simulink model "NL_valve"  (Simulink 7.8)
settings: Solver=ode45  StartTime=0.0  StopTime=time_span  RelTol=1e-3
values from neighbouring files (symbols this model uses):
  Cm = 5    [MSA_Controller.m]    (also in MSA_Controller_NL_valve.m = 1)
  par = [0.1,0.1,0.1]    [MSA_Controller.m]    (also in MSA_Controller_NL_valve.m = [0.1,0.1])
  samp_time = p.simulation.samp_time    [MSA_Controller.m]    (also in MSA_Controller_NL_valve.m)
libraries: simulink x1, simulink_need_slupdate x1
settings Model: Creator=KushalSahare  LastModifiedBy=KushalSahare

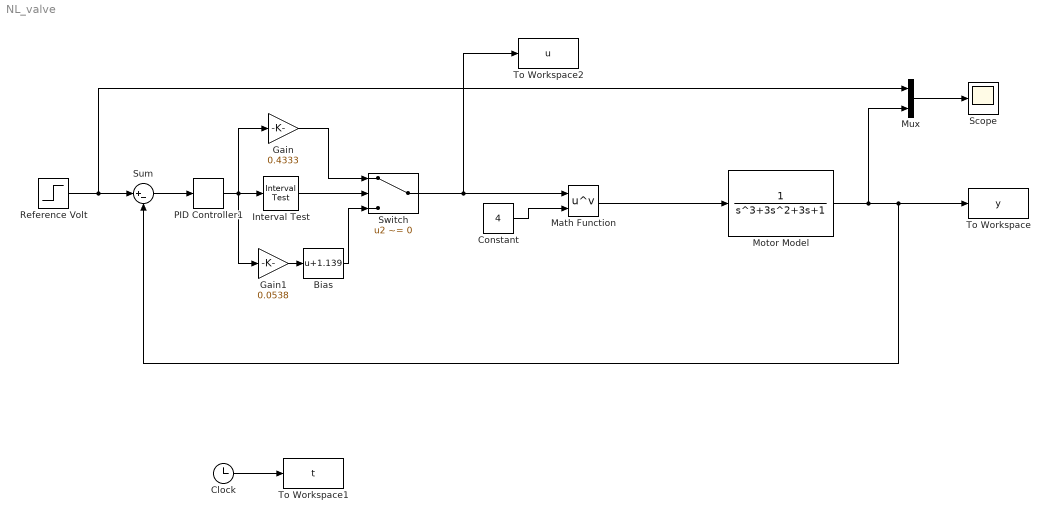
== system NL_valve ==
  Bias : Bias  Bias=1.139
  Clock : Clock
  Constant : Constant  Value=4
  Gain : Gain  Gain=0.4333
  Gain1 : Gain  Gain=0.0538
  Interval Test : simulink/Logic and Bit Operations/Interval Test  IntervalClosedRight=on  uplimit=3  IntervalClosedLeft=on  lowlimit=0  OutDataTypeStr=boolean
  Math Function : Math  Operator=pow  SaturateOnIntegerOverflow=on
  Motor Model : TransferFcn  Numerator=1  Denominator=[1, 3, 3, 1]
  Mux : Mux  Inputs=2
  PID Controller1 : simulink_need_slupdate/PID Controller  P=par(1)  I=par(2)  D=par(3)
  Reference Volt : Step  Time=0  After=Cm  SampleTime=0
  Scope : Scope
  Sum : Sum  Inputs=|+-
  Switch : Switch  Criteria=u2 ~= 0
  To Workspace : ToWorkspace  VariableName=y  SampleTime=samp_time  SaveFormat=Array
  To Workspace1 : ToWorkspace  VariableName=t  SampleTime=samp_time  SaveFormat=Array
  To Workspace2 : ToWorkspace  VariableName=u  SampleTime=samp_time  SaveFormat=Array
  wires:
  Motor Model/1 -> Sum/2, To Workspace/1, Mux/2
  Sum/1 -> PID Controller1/1
  PID Controller1/1 -> Interval Test/1, Gain/1, Gain1/1
  Reference Volt/1 -> Sum/1, Mux/1
  Constant/1 -> Math Function/2
  Math Function/1 -> Motor Model/1
  Clock/1 -> To Workspace1/1
  Mux/1 -> Scope/1
  Interval Test/1 -> Switch/2
  Switch/1 -> Math Function/1, To Workspace2/1
  Gain/1 -> Switch/1
  Gain1/1 -> Bias/1
  Bias/1 -> Switch/3
